simulink model "mpc1"  (R2020b)
settings: Solver=VariableStepAuto  StartTime=0.0  StopTime=48  RelTol=1e-3
libraries: mpclib x1, cstblocks x1, dspsrcs4 x1
settings Model: Creator=yanis  LastModifiedBy=yanis

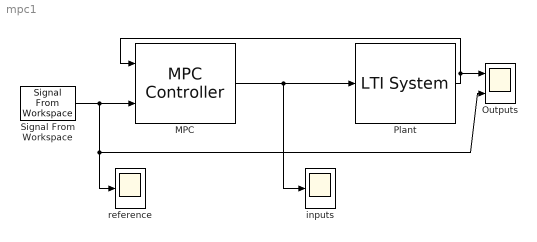
== system mpc1 ==
  MPC : mpclib/MPC Controller  SCDEnableBlockLinearizationSpecification=on  mpcobj=mpc1_C  is_multiple=0  enable_value=0  return_u0=off  updateMPCinCallerWorkspace=on  md_inport=off  mv_inport=off  uref_inport=off  return_cost=off  return_mvseq=off  return_qpstatus=off  return_xseq=off  return_state=off  return_ovseq=off  state_inport=off  umin_inport=off  umax_inport=off  ymin_inport=off  ymax_inport=off  cc_inport=off  ywt_inport=off  uwt_inport=off  duwt_inport=off  rhoeps_inport=off  pm_inport=off  MaximumP=10  HorizonChoice=FixedHorizon  n_ts=1  n_p=4  n_mv=2  n_md=0  n_ud=0  n_mo=2  n_uo=0  BlockDataType=double  SampleTimeInherited=off  switch_inport=off
  Outputs : Scope  NumInputPorts=2
  Plant : cstblocks/LTI System  sys=mpc1_G  IC=[]
  Signal From Workspace : dspsrcs4/Signal From Workspace  X=r  Ts=1  nsamps=1  OutputAfterFinalValue=Setting to zero  ignoreOrWarnInputAndFrameLengths=off  OutputFrames=off
  inputs : Scope
  reference : Scope
  wires:
  Signal From Workspace/1 -> Outputs/2, reference/1, MPC/2
  Plant/1 -> MPC/1, Outputs/1
  MPC/1 -> inputs/1, Plant/1
